simulink library "snippetLibrary"  (R2018a)
settings: Solver=VariableStepAuto  StartTime=0.0  StopTime=10.0  RelTol=1e-3
undefined symbols (not defined in the file): Aref
libraries: $bdroot x1, sharedutil x1
settings Model: Creator=Manit  LastModifiedBy=Manit

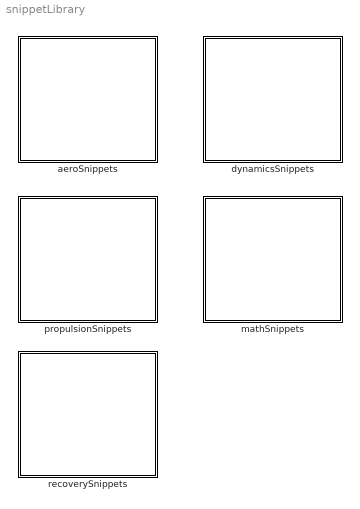
== system snippetLibrary ==
  aeroSnippets : Subsystem
  dynamicsSnippets : Subsystem
  mathSnippets : Subsystem
  propulsionSnippets : Subsystem
  recoverySnippets : Subsystem

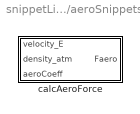
== system snippetLibrary/aeroSnippets ==
  calcAeroForce : Subsystem  mask{Aref=Aref}

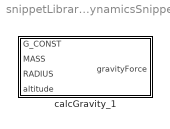
== system snippetLibrary/dynamicsSnippets ==
  calcGravity_1 : Subsystem

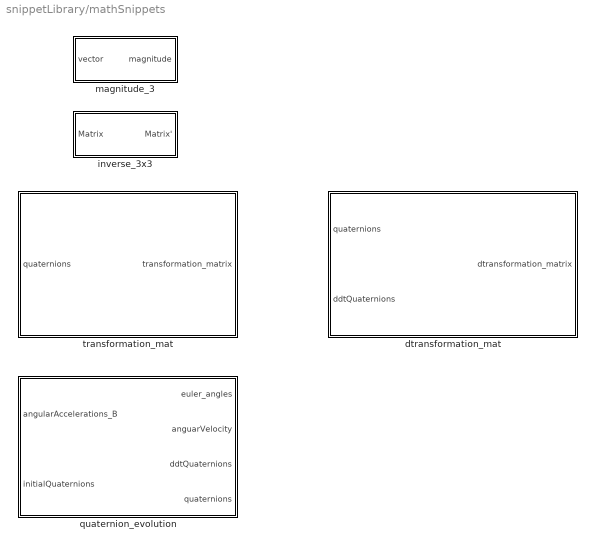
== system snippetLibrary/mathSnippets ==
  dtransformation_mat : MATLAB Function  TreatAsAtomicUnit=on
  inverse_3x3 : Subsystem
  magnitude_3 : Subsystem
  quaternion_evolution : Subsystem
  transformation_mat : MATLAB Function  TreatAsAtomicUnit=on

== system snippetLibrary/propulsionSnippets ==

== system snippetLibrary/recoverySnippets ==

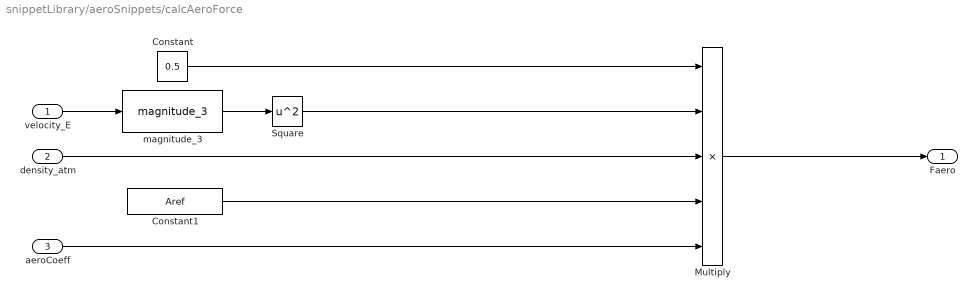
== system snippetLibrary/aeroSnippets/calcAeroForce ==
  velocity_E : Inport
  density_atm : Inport  Port=2
  aeroCoeff : Inport  Port=3
  Constant : Constant  Value=0.5
  Constant1 : Constant  Value=Aref
  Multiply : Product  Inputs=5
  Square : Math  Operator=square  SaturateOnIntegerOverflow=on
  magnitude_3 : $bdroot/mathSnippets/magnitude_3
  Faero : Outport
  wires:
  velocity_E/1 -> magnitude_3/1
  magnitude_3/1 -> Square/1
  Multiply/1 -> Faero/1
  Square/1 -> Multiply/2
  density_atm/1 -> Multiply/3
  Constant/1 -> Multiply/1
  aeroCoeff/1 -> Multiply/5
  Constant1/1 -> Multiply/4

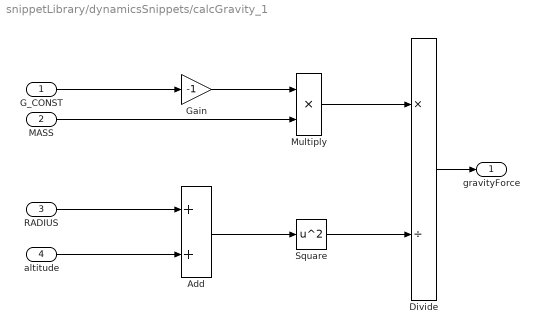
== system snippetLibrary/dynamicsSnippets/calcGravity_1 ==
  G_CONST : Inport
  MASS : Inport  Port=2
  RADIUS : Inport  Port=3
  altitude : Inport  Port=4
  Add : Sum
  Divide : Product  Inputs=*/
  Gain : Gain  Gain=-1
  Multiply : Product
  Square : Math  Operator=square  SaturateOnIntegerOverflow=on
  gravityForce : Outport
  wires:
  Divide/1 -> gravityForce/1
  G_CONST/1 -> Gain/1
  Multiply/1 -> Divide/1
  MASS/1 -> Multiply/2
  Gain/1 -> Multiply/1
  Square/1 -> Divide/2
  Add/1 -> Square/1
  altitude/1 -> Add/2
  RADIUS/1 -> Add/1

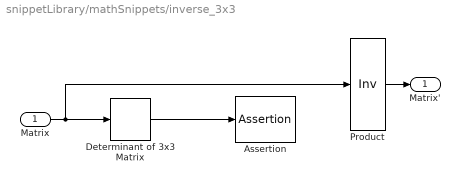
== system snippetLibrary/mathSnippets/inverse_3x3 ==
  Matrix : Inport  PortDimensions=[3 3]
  Assertion : Assertion  AssertionFailFcn="disp('Matrix is singular.  No matrix inverse.')"
  Determinant of 3x3 Matrix : sharedutil/Determinant of 3x3 Matrix  aMode=aMode
      settings: SourceProductName=Aerospace Blockset  SourceProductBaseCode=AE
  Product : Product  Inputs=/  Multiplication=Matrix(*)  SaturateOnIntegerOverflow=on  OutDataTypeStr=Inherit: Same as first input
  Matrix' : Outport  PortDimensions=[3 3]
  wires:
  Matrix/1 -> Product/1, Determinant of 3x3 Matrix/1
  Determinant of 3x3 Matrix/1 -> Assertion/1
  Product/1 -> Matrix'/1

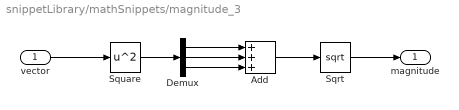
== system snippetLibrary/mathSnippets/magnitude_3 ==
  vector : Inport
  Add : Sum  Inputs=3
  Demux : Demux  Outputs=3
  Sqrt : Sqrt  SaturateOnIntegerOverflow=on
  Square : Math  Operator=square  SaturateOnIntegerOverflow=on
  magnitude : Outport
  wires:
  vector/1 -> Square/1
  Square/1 -> Demux/1
  Demux/1 -> Add/1
  Demux/2 -> Add/2
  Demux/3 -> Add/3
  Add/1 -> Sqrt/1
  Sqrt/1 -> magnitude/1

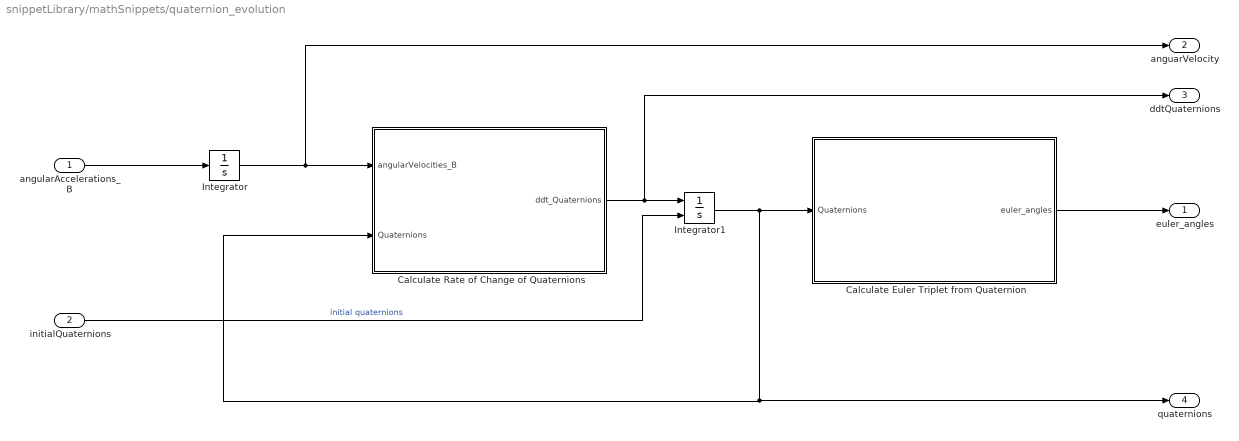
== system snippetLibrary/mathSnippets/quaternion_evolution ==
  angularAccelerations_B : Inport
  initialQuaternions : Inport  Port=2
  Calculate Euler Triplet from Quaternion : MATLAB Function  TreatAsAtomicUnit=on
  Calculate Rate of Change of Quaternions : MATLAB Function  TreatAsAtomicUnit=on
  Integrator : Integrator  InitialCondition=[0;0;0]
  Integrator1 : Integrator  InitialConditionSource=external  InitialCondition=[1;1;1;1]
  euler_angles : Outport
  anguarVelocity : Outport  Port=2
  ddtQuaternions : Outport  Port=3
  quaternions : Outport  Port=4
  wires:
  Integrator/1 -> anguarVelocity/1, Calculate Rate of Change of Quaternions/1(angularVelocities_B)
  angularAccelerations_B/1 -> Integrator/1
  Integrator1/1 -> quaternions/1, Calculate Rate of Change of Quaternions/2(Quaternions), Calculate Euler Triplet from Quaternion/1(Quaternions)
  initialQuaternions/1 -> Integrator1/2  "initial quaternions"
  Calculate Rate of Change of Quaternions/1(ddt_Quaternions) -> Integrator1/1, ddtQuaternions/1
  Calculate Euler Triplet from Quaternion/1(euler_angles) -> euler_angles/1

== matlab function snippetLibrary/mathSnippets/dtransformation_mat ==
  data: quaternions input; dtransformation_matrix output; ddtQuaternions input
function dtransformation_matrix = create_dtransformation_mat(quaternions, ddtQuaternions)

%q0 <=> quaternions(1);
%q1 <=> quaternions(2);
%q2 <=> quaternions(3);
%q3 <=> quaternions(4);

%dq0 <=> ddtQuaternions(1);
%dq1 <=> ddtQuaternions(2);
%dq2 <=> ddtQuaternions(3);
%dq3 <=> ddtQuaternions(4);

q0dq0_2 = 2*quaternions(1)*ddtQuaternions(1);
q1dq1_2 = 2*quaternions(2)*ddtQuaternions(2);
q2dq2_2 = 2*quaternions(3)*ddtQuaternions(3);
q3dq3_2 = 2*quaternions(4)*ddtQuaternions(4);

dq0q1 = ddtQuaternions(1)*quaternions(2);
q0dq1 = quaternions(1)*ddtQuaternions(2);

dq0q2 = ddtQuaternions(1)*quaternions(3);
q0dq2 = quaternions(1)*ddtQuaternions(3);

dq0q3 = ddtQuaternions(1)*quaternions(4);
q0dq3 = quaternions(1)*ddtQuaternions(4);

dq1q2 = ddtQuaternions(2)*quaternions(3);
q1dq2 = quaternions(2)*ddtQuaternions(3);

dq1q3 = ddtQuaternions(2)*quaternions(4);
q1dq3 = quaternions(2)*ddtQuaternions(4);

dq2q3 = ddtQuaternions(3)*quaternions(4);
q2dq3 = quaternions(3)*ddtQuaternions(4);

dtransformation_matrix = [(q0dq0_2 + q1dq1_2 - q2dq2_2 - q3dq3_2)  2*(dq1q2 + q1dq2 - (dq0q3 + q0dq3))      2*(dq0q2 + q0dq2 + dq1q3+q1dq3);
                          2*(dq1q2 + q1dq2 + dq0q3 + q0dq3)        (q0dq0_2 - q1dq1_2 + q2dq2_2 - q3dq3_2)  2*(dq2q3 + q2dq3 - (dq0q1 + q0dq1));
                          2*(dq1q3 + q1dq3 - (dq0q2 + q0dq2))      2*(dq0q1 + q0dq1 + dq2q3 + q2dq3)        (q0dq0_2 - q1dq1_2 - q2dq2_2 + q3dq3_2)];

== matlab function snippetLibrary/mathSnippets/quaternion_evolution/Calculate Rate of Change of Quaternions ==
  data: angularVelocities_B input; ddt_Quaternions output; Quaternions input
function ddt_Quaternions = ddtQuaternions(angularVelocities_B, Quaternions)


p = angularVelocities_B(1);
q = angularVelocities_B(2);
r = angularVelocities_B(3);

qT = [0 -p -q -r; p 0 r -q; q -r 0 p; r q -p 0];

ddt_Quaternions = 0.5*qT*Quaternions;

== matlab function snippetLibrary/mathSnippets/quaternion_evolution/Calculate Euler Triplet from Quaternion ==
  data: Quaternions input; euler_angles output
function euler_angles = qToEuler(Quaternions)

q0 = Quaternions(1);
q1 = Quaternions(2);
q2 = Quaternions(3);
q3 = Quaternions(4);

Phi = atan2(2.*(q0.*q1 + q2.*q3), 1 - 2.*(q1^2 + q2^2));
Theta = asin(2.*(q0.*q2 - q3.*q1));
Psi = atan2(2.*(q0.*q3 +q1.*q2), 1 - 2.*(q2^2 + q3^2));

euler_angles = [Phi; Theta; Psi];

== matlab function snippetLibrary/mathSnippets/transformation_mat ==
  data: quaternions input; transformation_matrix output
function transformation_matrix = create_transformation_mat(quaternions)

%q0 <=> quaternions(1);
%q1 <=> quaternions(2);
%q2 <=> quaternions(3);
%q3 <=> quaternions(4);

q0_sq = quaternions(1)^2;
q1_sq = quaternions(2)^2;
q2_sq = quaternions(3)^2;
q3_sq = quaternions(4)^2;

q0q1 = quaternions(1)*quaternions(2);
q0q2 = quaternions(1)*quaternions(3);
q0q3 = quaternions(1)*quaternions(4);
q1q2 = quaternions(2)*quaternions(3);
q1q3 = quaternions(2)*quaternions(4);
q2q3 = quaternions(3)*quaternions(4);

transformation_matrix = [ (q0_sq + q1_sq - q2_sq - q3_sq)  2*(q1q2-q0q3)                    2*(q0q2+q1q3);
                          2*(q1q2+q0q3)                    (q0_sq - q1_sq + q2_sq - q3_sq)  2*(q2q3-q0q1);
                          2*(q1q3-q0q2)                    2*(q0q1+q2q3)                    (q0_sq - q1_sq - q2_sq + q3_sq)];
